simulink model "sldemo_househeat_non_linear"  (R2024b)
settings: Solver=ode4  StartTime=0.0  StopTime=604800  FixedStep=60  RelTol=1e-3  AbsTol=1e-6
model workspace (MATLAB code in the model file):
  | % load initial conditions and physical properties from file
  | 
  | sldemo_househeat_data
undefined symbols (not defined in the file): alpha, c_air, cbrick, cost, epsilon, Ki, Kp, M_air, Mbrick, QAerotermia, R0, roofArea, sigma, TinIC
libraries: slpidlib x1, thermostat x1
Description:
  | Thermal Model of a House
  | 
  | This demo illustrates how you can use Simulink(R) to create the thermal model of
  | a house. This system models the outdoor environment, the thermal
  | characteristics of the house, and the house heating system.
  | 
  | The sldemo_househeat_data.m file initializes data in the model workspace.
  | To make changes, you can edit the model workspace directly or edit the MATLAB(R) file
  | and re-load the model workspace.
  | 
  | To view the model workspace, select View > Model Explorer
  | from the Simulink editor.
  | 
  | Note: Time is given in units of hours
settings Model: Creator=The MathWorks, Inc.  LastModifiedBy=fergusproctor
settings SolverCC: AutoScaleAbsTol=off  AlgebraicLoopSolver=TrustRegion
settings DataIOCC: ExternalInput=[]  InitialState=[]
settings OptimizationCC: BlockReduction=off  BooleanDataType=off  ReuseModelBlockBuffer=off  ExpressionDepthLimit=2147483647  InitFltsAndDblsToZero=on  LifeSpan=inf  BufferReusableBoundary=off
settings DebuggingCC: SaveWithParameterizedLinksMsg=none  UnderspecifiedInitializationDetection=Classic  MergeDetectMultiDrivingBlocksExec=none  SignalResolutionControl=TryResolveAllWithWarning  MultiTaskDSMMsg=warning  MultiTaskCondExecSysMsg=none  IntegerOverflowMsg=none  FcnCallInpInsideContextMsg=warning  UnconnectedInputMsg=warning  UnconnectedOutputMsg=warning  UnconnectedLineMsg=warning  BusObjectLabelMismatch=none  StateNameClashWarn=warning  SFUnexpectedBacktrackingDiag=warning  SFNoUnconditionalDefaultTransitionDiag=warning  SFExecutionAtInitializationDiag=none  IntegerSaturationMsg=none  ArithmeticOperatorsInVariantConditions=warning
settings HardwareCC: ProdBitPerPointer=32  ProdBitPerSizeT=32  ProdBitPerPtrDiffT=32  ProdLargestAtomicFloat=None  ProdIntDivRoundTo=Undefined  ProdEndianess=Unspecified  ProdWordSize=32  ProdHWDeviceType=32-bit Generic  TargetUnknown=on
settings ModelReferenceCC: EnableRefExpFcnMdlSchedulingChecks=on  PropagateSignalLabelsOutOfModel=off
settings SFSimCC: SimUseLocalCustomCode=off  CustomCodeUndefinedFunction=UseInterfaceOnly
settings RTWCC: RTWUseLocalCustomCode=off  GPUComputeCapability=3.5
settings CodeAppCC: StateflowObjectComments=on
settings GRTTargetCC: TargetFcnLib=ansi_tfl_tmw.mat  TargetLangStandard=C89/C90 (ANSI)  CombineOutputUpdateFcns=off  GRTInterface=on
settings ConfigComp: CovMetricSettings=dw  CovSaveCumulativeToWorkspaceVar=on  CovSaveSingleToWorkspaceVar=on  CovExternalEMLEnable=off

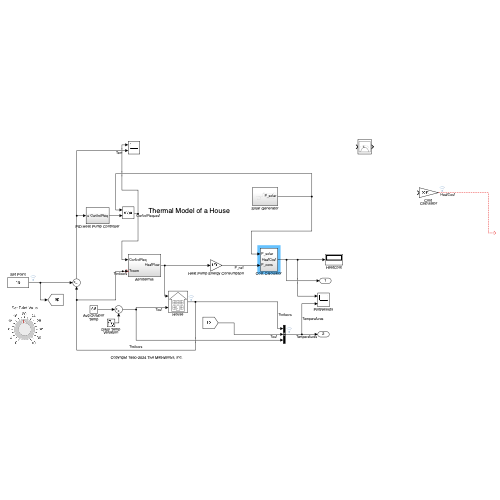
[thumbnail: Simulink's stored preview of the top-level diagram]
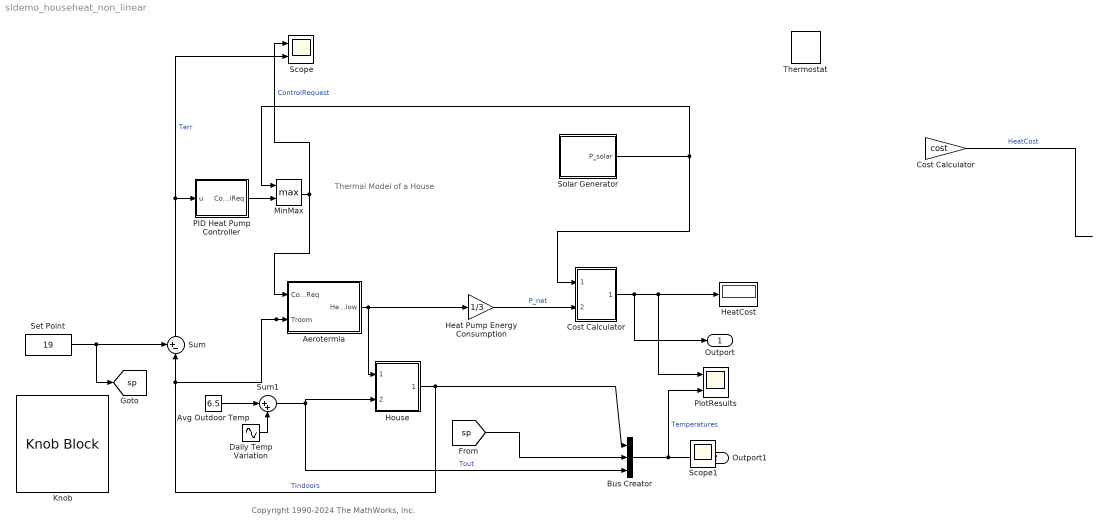
== system sldemo_househeat_non_linear ==
  note: Thermal Model of a House
  note: Copyright 1990-2024 The MathWorks, Inc.
  Aerotermia : Subsystem
  Avg Outdoor Temp : Constant  Value=6.5
  Bus Creator : BusCreator  Inputs=3
  Cost Calculator : Gain  Gain=cost  SaturateOnIntegerOverflow=on  OutDataTypeStr=Inherit: Same as input  ParamDataTypeStr=Inherit: Same as input
  Cost Calculator : Subsystem
  Daily Temp Variation : Sin  Amplitude=3.5  Frequency=(2*pi)/(24*3600)  SampleTime=0
  Heat Pump Energy Consumption : Gain  Gain=1/3
  HeatCost : Display
  House : Subsystem
      mask Display: image('HouseHeatHousePix.svg')
  Knob : KnobBlock  ScaleMax=40
  MinMax : MinMax  Function=max  Inputs=2
  PID Heat Pump Controller : Subsystem
  PlotResults : Scope  NumInputPorts=2
  Scope : Scope  NumInputPorts=2
  Set Point : Constant  Value=19
  Solar Generator : Subsystem
  Sum : Sum  Inputs=+-|  InputSameDT=on  SaturateOnIntegerOverflow=on  OutDataTypeStr=Inherit: Same as first input
  Sum1 : Sum  Inputs=|++  InputSameDT=on  SaturateOnIntegerOverflow=on  OutDataTypeStr=Inherit: Same as first input
  Thermostat : thermostat/Thermostat  SystemSampleTime=-1  VariantActivationTime=update diagram  AllowFlexibleInterface=on  Latency=0  AutoFrameSizeCalculation=off
  Outport : Outport
  Outport1 : Outport  Port=2
  Scope1 : Scope
  tag scope: sp=global
  wires:
  Aerotermia/1(HeatFlow) -> Heat Pump Energy Consumption/1, House/1(Heater QDot In)
  Sum/1 -> Scope/2, PID Heat Pump Controller/1(u)  "Terr"
  Daily Temp Variation/1 -> Sum1/2
  Avg Outdoor Temp/1 -> Sum1/1
  House/1(Room Temp Troom) -> Bus Creator/1, Aerotermia/2(Troom), Sum/2  "Tindoors"
  Sum1/1 -> House/2(Outdoor Temp Tout), Bus Creator/3  "Tout"
  Bus Creator/1 -> Outport1/1, PlotResults/2  "Temperatures"
  Set Point/1 -> [sp], Sum/1
  [sp] -> Bus Creator/2
  Heat Pump Energy Consumption/1 -> Cost Calculator/2(P_cons)  "P_net"
  Cost Calculator/1(HeatCost) -> Outport/1, PlotResults/1, HeatCost/1
  Solar Generator/1(P_solar) -> MinMax/1, Cost Calculator/1(P_solar)
  Cost Calculator/1 -> ?  "HeatCost"
  PID Heat Pump Controller/1(ControlReq) -> MinMax/2
  MinMax/1 -> Scope/1, Aerotermia/1(ControlReq)  "ControlRequest"

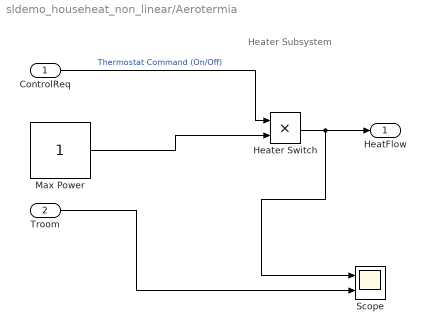
== system sldemo_househeat_non_linear/Aerotermia ==
  note: Heater Subsystem
  ControlReq : Inport
  Troom : Inport  Port=2
  Heater Switch : Product  RndMeth=Zero
  Max Power : Constant
  Scope : Scope  NumInputPorts=2
  HeatFlow : Outport  VectorParamsAs1DForOutWhenUnconnected=off
  wires:
  ControlReq/1 -> Heater Switch/1  "Thermostat Command (On/Off)"
  Max Power/1 -> Heater Switch/2
  Heater Switch/1 -> Scope/1, HeatFlow/1
  Troom/1 -> Scope/2

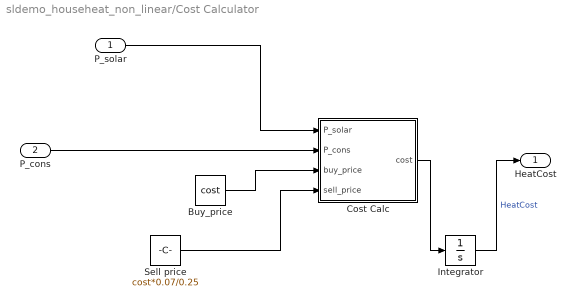
== system sldemo_househeat_non_linear/Cost Calculator ==
  P_solar : Inport
  P_cons : Inport  Port=2
  Buy_price : Constant  Value=cost
  Cost Calc : MATLAB Function  TreatAsAtomicUnit=on
  Integrator : Integrator
  Sell price : Constant  Value=cost*0.07/0.25
  HeatCost : Outport
  wires:
  Cost Calc/1(cost) -> Integrator/1
  P_solar/1 -> Cost Calc/1(P_solar)
  Buy_price/1 -> Cost Calc/3(buy_price)
  P_cons/1 -> Cost Calc/2(P_cons)
  Sell price/1 -> Cost Calc/4(sell_price)
  Integrator/1 -> HeatCost/1  "HeatCost"

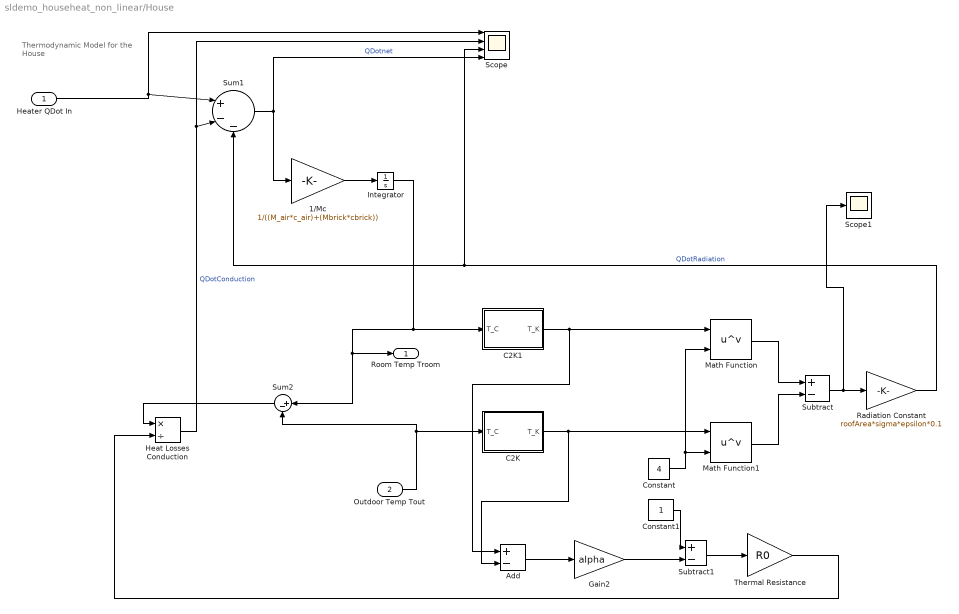
== system sldemo_househeat_non_linear/House ==
  note: Thermodynamic Model
      | for the House
  Heater QDot In : Inport
  Outdoor Temp Tout : Inport  Port=2
  1/Mc : Gain  Gain=1/((M_air*c_air)+(Mbrick*cbrick))  SaturateOnIntegerOverflow=on  OutDataTypeStr=Inherit: Same as input  ParamDataTypeStr=Inherit: Same as input
  Add : Sum  Inputs=+-
  C2K : MATLAB Function  TreatAsAtomicUnit=on
  C2K1 : MATLAB Function  TreatAsAtomicUnit=on
  Constant : Constant  Value=4
  Constant1 : Constant
  Gain2 : Gain  Gain=alpha
  Heat Losses Conduction : Product  Inputs=*/
  Integrator : Integrator  InitialCondition=TinIC
  Math Function : Math  Operator=pow
  Math Function1 : Math  Operator=pow
  Radiation Constant : Gain  Gain=roofArea*sigma*epsilon*0.1
  Scope : Scope  NumInputPorts=4
  Scope1 : Scope
  Subtract : Sum  Inputs=+-
  Subtract1 : Sum  Inputs=+-
  Sum1 : Sum  Inputs=|+--  InputSameDT=on  SaturateOnIntegerOverflow=on  OutDataTypeStr=Inherit: Same as first input
  Sum2 : Sum  Inputs=|+-  InputSameDT=on  SaturateOnIntegerOverflow=on  OutDataTypeStr=Inherit: Same as first input
  Thermal Resistance : Gain  Gain=R0
  Room Temp Troom : Outport  InitialOutput=0  VectorParamsAs1DForOutWhenUnconnected=off
  wires:
  Outdoor Temp Tout/1 -> Sum2/2, C2K/1(T_C)
  Heater QDot In/1 -> Scope/1, Sum1/1
  Sum1/1 -> 1/Mc/1, Scope/4  "QDotnet"
  Sum2/1 -> Heat Losses Conduction/1
  1/Mc/1 -> Integrator/1
  Integrator/1 -> Room Temp Troom/1, Sum2/1, C2K1/1(T_C)
  C2K1/1(T_K) -> Add/1, Math Function/1
  C2K/1(T_K) -> Add/2, Math Function1/1
  Constant/1 -> Math Function/2, Math Function1/2
  Math Function/1 -> Subtract/1
  Math Function1/1 -> Subtract/2
  Subtract/1 -> Scope1/1, Radiation Constant/1
  Constant1/1 -> Subtract1/1
  Gain2/1 -> Subtract1/2
  Add/1 -> Gain2/1
  Thermal Resistance/1 -> Heat Losses Conduction/2
  Heat Losses Conduction/1 -> Scope/2, Sum1/2  "QDotConduction"
  Radiation Constant/1 -> Scope/3, Sum1/3  "QDotRadiation"
  Subtract1/1 -> Thermal Resistance/1

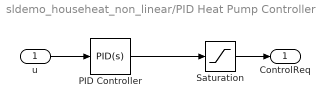
== system sldemo_househeat_non_linear/PID Heat Pump Controller ==
  u : Inport
  PID Controller : slpidlib/PID Controller  Controller=PID  Form=Parallel  TimeDomain=Continuous-time  UseExternalTs=off  SampleTime=-1  IntegratorMethod=Forward Euler  FilterMethod=Forward Euler  ControllerParametersSource=internal  P=Kp  I=Ki  UseKiTs=off  D=0  UseExternalDerivativeSource=off  N=4  UseFilter=on  TunerSelectOption=Transfer Function Based (PID Tuner App)  InitialConditionSource=internal  InitialConditionForIntegrator=0  InitialConditionForFilter=0  DifferentiatorICPrevScaledInput=0  ExternalReset=none  TrackingMode=off  Kt=1  LimitOutput=off  SatLimitsSource=internal  UpperSaturationLimit=inf  LowerSaturationLimit=-inf  LinearizeAsGain=on  AntiWindupMode=none  Kb=1  LimitIntegrator=off  UpperIntegratorSaturationLimit=inf  LowerIntegratorSaturationLimit=-inf  POutMin=[]  POutMax=[]  IOutMin=[]  IOutMax=[]  DOutMin=[]  DOutMax=[]  NOutMin=[]  NOutMax=[]  SumOutMin=[]  SumOutMax=[]  SaturationOutMin=[]  SaturationOutMax=[]  PParamMin=[]  PParamMax=[]  IParamMin=[]  IParamMax=[]  DParamMin=[]  DParamMax=[]  NParamMin=[]  NParamMax=[]  KbParamMin=[]  KbParamMax=[]  KtParamMin=[]  KtParamMax=[]  KbOutMin=[]  KbOutMax=[]  KtOutMin=[]  KtOutMax=[]  IntegratorOutMin=[]  IntegratorOutMax=[]  FilterOutMin=[]  FilterOutMax=[]  SumI1OutMin=[]  SumI1OutMax=[]  SumI2OutMin=[]  SumI2OutMax=[]  SumI3OutMin=[]  SumI3OutMax=[]  SumI4OutMin=[]  SumI4OutMax=[]  SumDOutMin=[]  SumDOutMax=[]  DifferentiatorOutMin=[]  DifferentiatorOutMax=[]  FilterDiffOutCoefMin=[]  FilterDiffOutCoefMax=[]  ReciprocalOutMin=[]  ReciprocalOutMax=[]  SumDenOutMin=[]  SumDenOutMax=[]  SumNumOutMin=[]  SumNumOutMax=[]  DivideOutMin=[]  DivideOutMax=[]  UdiffTsProdOutMin=[]  UdiffTsProdOutMax=[]  NTsProdOutMin=[]  NTsProdOutMax=[]  UintegralTsProdOutMin=[]  UintegralTsProdOutMax=[]  UngainTsProdOutMin=[]  UngainTsProdOutMax=[]  ClampingZeroOutDataTypeStr=Inherit: Inherit via back propagation  ClampingZeroOutMin=[]  ClampingZeroOutMax=[]  FilterDenConstantOutDataTypeStr=Inherit: Inherit via back propagation  FilterDenConstantOutMin=[]  FilterDenConstantOutMax=[]  PCopyOutDataTypeStr=Inherit: Inherit via back propagation  PCopyOutMin=[]  PCopyOutMax=[]  NCopyOutDataTypeStr=Inherit: Inherit via back propagation  NCopyOutMin=[]  NCopyOutMax=[]  IntegratorContinuousStateAttributes=''  IntegratorStateMustResolveToSignalObject=off  IntegratorRTWStateStorageClass=Auto  FilterContinuousStateAttributes=''  FilterStateMustResolveToSignalObject=off  FilterRTWStateStorageClass=Auto  ParallelPVariant=InternalParameters  IdealPVariant=Disabled  IVariant=InternalParameters  DVariant=InternalParameters  IntegratorVariant=Continuous  SatVariant=Disabled  AWVariant=Passthrough  PCopyVariant=Disabled  TRVariant=Disabled  FdbkBlocksVariant=Forward  IdealPFdbkVariant=Disabled  SatFdbkVariant=Disabled  DerivativeFilterVariant=ContFilter  NVariant=InternalParameters  NCopyVariant=Disabled  FilterICVariant=InternalICsFilter  IntegratorICVariant=InternalICs  ExternalResetVariant=Disabled  TRSumVariant=Passthrough  SumFdbkVariant=Disabled  SumVariant=Sum_PID  TsampFilterVariant=InternalTs  TsampNgainVariant=Passthrough  TsampIntegralVariant=Disabled_SignalSpec  ExternalSaturationOutDataTypeStr=Inherit: Same as second input  DerivativeSourceVariant=ErrorSignal  PreIntVariant=InternalPreInt
  Saturation : Saturate  UpperLimit=QAerotermia  LowerLimit=0
  ControlReq : Outport
  wires:
  u/1 -> PID Controller/1
  PID Controller/1 -> Saturation/1
  Saturation/1 -> ControlReq/1

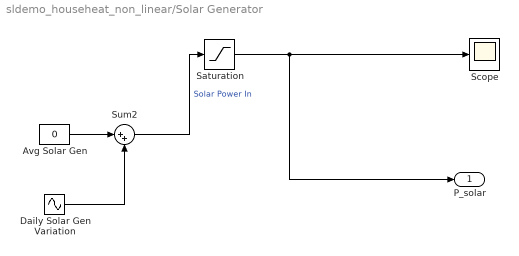
== system sldemo_househeat_non_linear/Solar Generator ==
  Avg Solar Gen : Constant  Value=0
  Daily Solar Gen Variation : Sin  Amplitude=2000  Frequency=(2*pi)/(24*3600)  SampleTime=0
  Saturation : Saturate  UpperLimit=inf  LowerLimit=0
  Scope : Scope
  Sum2 : Sum  Inputs=|++  InputSameDT=on  SaturateOnIntegerOverflow=on  OutDataTypeStr=Inherit: Same as first input
  P_solar : Outport
  wires:
  Daily Solar Gen Variation/1 -> Sum2/2
  Avg Solar Gen/1 -> Sum2/1
  Sum2/1 -> Saturation/1  "Solar Power In"
  Saturation/1 -> P_solar/1, Scope/1

== matlab function sldemo_househeat_non_linear/House/C2K1 ==
  data: T_C input; T_K output



function T_K = celsiusToKelvin(T_C)
T_K = T_C + 273.15;
end

== matlab function sldemo_househeat_non_linear/House/C2K ==
  data: T_C input; T_K output



function T_K = celsiusToKelvin(T_C)
T_K = T_C + 273.15;
end

== matlab function sldemo_househeat_non_linear/Cost Calculator/Cost Calc ==
  data: P_solar input; cost output; P_cons input; buy_price input; sell_price input
function cost = gridCost(P_solar, P_cons, buy_price, sell_price)
P_net =   P_cons - P_solar;
if P_net >= 0
    cost = P_net * buy_price;
else
    cost = P_net * sell_price;
end
end
